simulink model "hf2simuAQCOKQ"  (R2023a)
settings: Solver=VariableStepAuto  StartTime=0.0  StopTime=10  RelTol=1e-3
values from neighbouring files (symbols this model uses):
  A = [0 1 0 0 ... (first row only)    [hf2AQCOKQ.m]
  B = [0 ... (first row only)    [hf2AQCOKQ.m]
  C = [1 0 0 0 ... (first row only)    [hf2AQCOKQ.m]
  D = zeros(2, 1)    [hf2AQCOKQ.m]
  kw1 = 2 * 10^4    (= 20000)    [hf2AQCOKQ.m]
  kw3 = -2 * 10^9    (= -2000000000)    [hf2AQCOKQ.m]
settings Model: Creator=simon  LastModifiedBy=simon

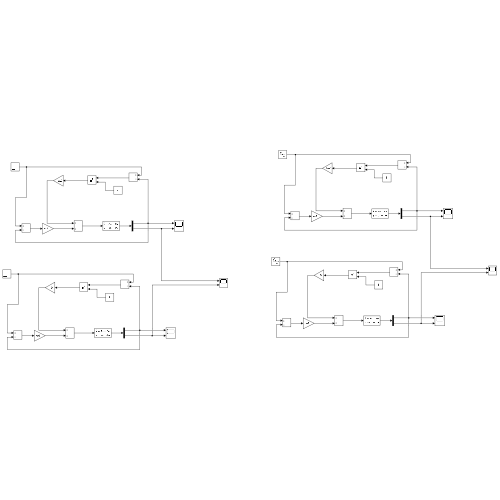
[thumbnail: Simulink's stored preview of the top-level diagram]
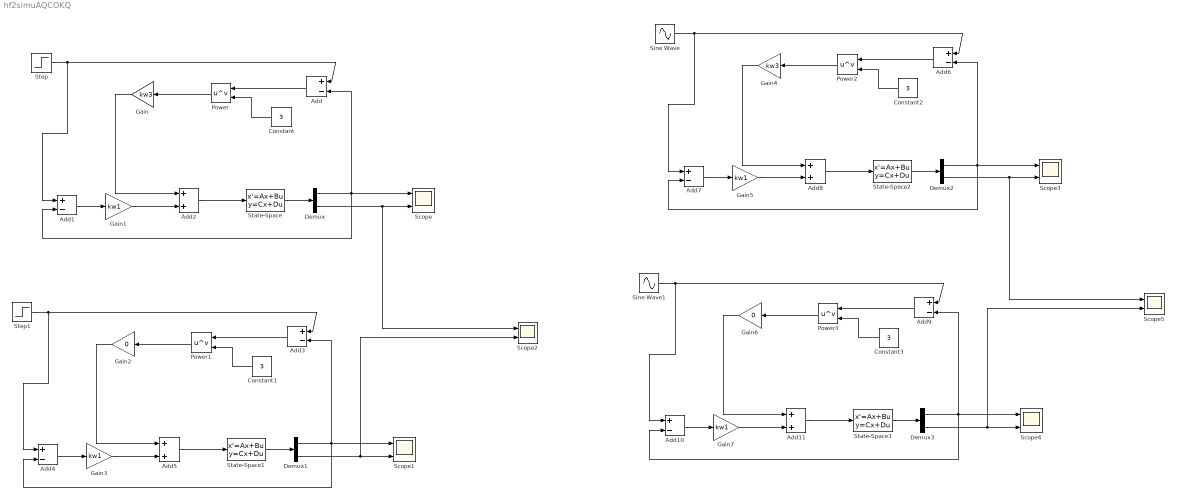
== system hf2simuAQCOKQ ==
  Add{,1,3..4,6..7,9..10} (8 alike) : Sum  Inputs=+-
  Add{2,5,8,11} (4 alike) : Sum
  Constant{,1..3} (4 alike) : Constant  Value=3
  Demux{,1..3} (4 alike) : Demux  Outputs=2
  Gain : Gain  Gain=kw3
  Gain{1,3,5,7} (4 alike) : Gain  Gain=kw1
  Gain2 : Gain  Gain=0
  Gain4 : Gain  Gain=kw3
  Gain6 : Gain  Gain=0
  Power{,1..3} (4 alike) : Math  Operator=pow
  Scope{,1..5} (6 alike) : Scope  NumInputPorts=2
  Sine Wave : Sin  Amplitude=0.01  SampleTime=0
  Sine Wave1 : Sin  Amplitude=0.01  SampleTime=0
  State-Space{,1..3} (4 alike) : StateSpace  A=A  B=B  C=C  D=D  InitialCondition=0
  Step : Step  After=0.001  OutDataTypeStr=single  SampleTime=0
  Step1 : Step  After=0.001  OutDataTypeStr=single  SampleTime=0
  wires:
  State-Space/1 -> Demux/1
  Demux/1 -> Add1/2, Add/2, Scope/1
  Demux/2 -> Scope2/1, Scope/2
  Step/1 -> Add1/1, Add/1
  Add/1 -> Power/1
  Constant/1 -> Power/2
  Power/1 -> Gain/1
  Gain/1 -> Add2/1
  Add2/1 -> State-Space/1
  Gain1/1 -> Add2/2
  Add1/1 -> Gain1/1
  Add4/1 -> Gain3/1
  Gain3/1 -> Add5/2
  Constant1/1 -> Power1/2
  Add5/1 -> State-Space1/1
  Gain2/1 -> Add5/1
  Step1/1 -> Add4/1, Add3/1
  Demux1/1 -> Add4/2, Add3/2, Scope1/1
  Power1/1 -> Gain2/1
  Add3/1 -> Power1/1
  Demux1/2 -> Scope2/2, Scope1/2
  State-Space1/1 -> Demux1/1
  State-Space3/1 -> Demux3/1
  Constant3/1 -> Power3/2
  Gain6/1 -> Add11/1
  Add9/1 -> Power3/1
  Demux3/1 -> Add10/2, Add9/2, Scope4/1
  Add11/1 -> State-Space3/1
  Power3/1 -> Gain6/1
  Add10/1 -> Gain7/1
  Add7/1 -> Gain5/1
  Gain5/1 -> Add8/2
  Constant2/1 -> Power2/2
  Add8/1 -> State-Space2/1
  Gain4/1 -> Add8/1
  Sine Wave/1 -> Add7/1, Add6/1
  Sine Wave1/1 -> Add10/1, Add9/1
  Demux2/1 -> Add7/2, Add6/2, Scope3/1
  Power2/1 -> Gain4/1
  Add6/1 -> Power2/1
  Demux2/2 -> Scope5/1, Scope3/2
  Gain7/1 -> Add11/2
  State-Space2/1 -> Demux2/1
  Demux3/2 -> Scope5/2, Scope4/2
